simulink model "plant1_noObserver"  (R2015a)
settings: Solver=ode45  StartTime=0.0  StopTime=10.0  RelTol=1e-3
values from neighbouring files (symbols this model uses):
  A = [2.15382349002 0.214572825654 1.88950096566 -0.29867853041 0.113062196229 -1.01325242733 0.619436209547 2.86203861181 4.48591725582 -0.687413149535 3.93984391159 1.51814076611 ... (36 elements, 6x6)]    [De2.mat]    (also in main_elca.m = [   -2.1     0.3     0.5     0.9; main_elca_nonsquare.m = [-31.31 0 -2.833e4;0 -10.25 8001;1 -1 0]; main_elca_siso.m = [-31.31 0 -2.833e4;0 -10.25 8001;1 -1 0]; main_elca_siso_conference.m = [-31.31 0 -2.833e4;0 -10.25 8001;1 -1 0])
  B = [-3.59754701628 1.03900107164 -0.0588288788819 1.91030576689 -0.469593029649 2.39038747798 -2.63971513379 2.37119746965 -0.382769327239 -1.07761123079 -0.524364953631 2.34772297005 ... (18 elements, 6x3)]    [De2.mat]    (also in main_elca.m = [   1   -0.4; main_elca_nonsquare.m = [28.06 0 0]'; main_elca_siso.m = [28.06 0 0]'; main_elca_siso_conference.m = [28.06;0;0])
  C = [2.23974909489  -2.89672334174  -0.970355173176  -2.60836731796  -0.958327072966  -1.82597470965; -0.233950036489  3.17111373121  -0.953917376412  0.311760155602  0.255404296822  2.81333280658]    [De2.mat]    (also in main_elca.m = [2  -2  -1   4; main_elca_nonsquare.m = [1 0 0]; main_elca_siso.m = [1 0 0]; main_elca_siso_conference.m = [1 0 0])
  D = [0  0  0; 0  0  0]    [De2.mat]    (also in main_c.m = zeros(p,m); main_elca.m = zeros(p,m); main_elca_nonsquare.m = zeros(p,m); main_elca_siso.m = zeros(p,m))
  Ec = -inv(R_bar)*( ( C - D*Kc )*inv( A - B*Kc )*B - D )'*Qc    [TZOCS.m]    (also in main_c.m = -inv(R_bar)*( ( C_aug - D_aug*Kc )*inv( A_aug - B_aug*Kc )*B; main_elca.m = -inv(R_bar)*( ( C_aug - D_aug*Kc )*inv( A_aug - B_aug*Kc )*B; main_elca_nonsquare.m = -inv(R_bar)*( ( C_aug - D_aug*Kc )*inv( A_aug - B_aug*Kc )*B; main_elca_siso.m = -inv(R_bar)*( ( C_aug - D_aug*Kc )*inv( A_aug - B_aug*Kc )*B)
  eta = 0.532094499421    [eta value.mat]    (also in eta_value.mat = [-2.43750362486  -7.92336865107; -8.9760065871  -9.529746909; generate_eta.m = (1*randn(p,p)); main_c.m = 10*eta; main_elca_nonsquare.m = eye(1))
  Kc1 = Kc(:,1:n)    [main_c.m]    (also in main_elca.m; main_elca_nonsquare.m; main_elca_siso.m; main_elca_siso_conference.m)
  Kc2 = Kc(:,n+1:end)    [main_c.m]    (also in main_elca.m; main_elca_nonsquare.m; main_elca_siso.m; main_elca_siso_conference.m)
  Kd_1 = Kd(1,1)    [main_c.m]    (also in main_elca.m; main_elca_nonsquare.m; main_elca_siso.m; main_elca_siso_conference.m)
  Ki_1 = Ki(1,1)    [main_c.m]    (also in main_elca.m; main_elca_nonsquare.m; main_elca_siso.m; main_elca_siso_conference.m)
  Kp_1 = Kp(1,1)    [main_c.m]    (also in main_elca.m; main_elca_nonsquare.m; main_elca_siso.m; main_elca_siso_conference.m)
settings Model: Creator=Elca  LastModifiedBy=Elca

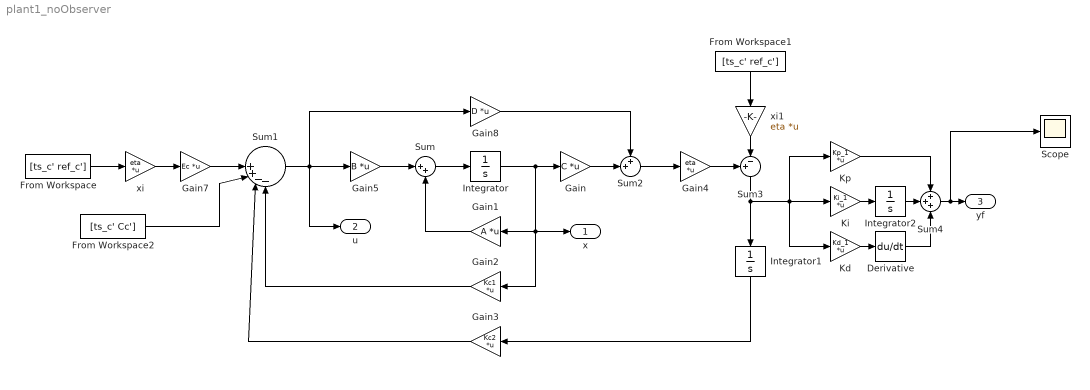
== system plant1_noObserver ==
  Derivative : Derivative
  From Workspace : FromWorkspace  VariableName=[ts_c' ref_c']  SampleTime=0
  From Workspace1 : FromWorkspace  VariableName=[ts_c' ref_c']  SampleTime=0
  From Workspace2 : FromWorkspace  VariableName=[ts_c' Cc']  SampleTime=0
  Gain : Gain  Gain=C  Multiplication=Matrix(K*u)
  Gain1 : Gain  Gain=A  Multiplication=Matrix(K*u)
  Gain2 : Gain  Gain=Kc1  Multiplication=Matrix(K*u)
  Gain3 : Gain  Gain=Kc2  Multiplication=Matrix(K*u)
  Gain4 : Gain  Gain=eta  Multiplication=Matrix(K*u)
  Gain5 : Gain  Gain=B  Multiplication=Matrix(K*u)
  Gain7 : Gain  Gain=Ec  Multiplication=Matrix(K*u)
  Gain8 : Gain  Gain=D  Multiplication=Matrix(K*u)
  Integrator : Integrator
  Integrator1 : Integrator
  Integrator2 : Integrator
  Kd : Gain  Gain=Kd_1  Multiplication=Matrix(K*u)
  Ki : Gain  Gain=Ki_1  Multiplication=Matrix(K*u)
  Kp : Gain  Gain=Kp_1  Multiplication=Matrix(K*u)
  Scope : Scope
  Sum : Sum  Inputs=|++
  Sum1 : Sum  Inputs=|||++--
  Sum2 : Sum  Inputs=++|
  Sum3 : Sum  Inputs=+-|
  Sum4 : Sum  Inputs=+++
  xi : Gain  Gain=eta  Multiplication=Matrix(K*u)
  xi1 : Gain  Gain=eta  Multiplication=Matrix(K*u)
  x : Outport
  u : Outport  Port=2
  yf : Outport  Port=3
  wires:
  Gain7/1 -> Sum1/1
  Integrator/1 -> Gain2/1, x/1, Gain1/1, Gain/1
  Sum2/1 -> Gain4/1
  Gain/1 -> Sum2/2
  Gain8/1 -> Sum2/1
  Sum1/1 -> Gain8/1, u/1, Gain5/1
  Sum/1 -> Integrator/1
  Gain1/1 -> Sum/2
  Gain5/1 -> Sum/1
  From Workspace/1 -> xi/1
  Integrator1/1 -> Gain3/1
  From Workspace2/1 -> Sum1/2
  Gain2/1 -> Sum1/4
  Gain3/1 -> Sum1/3
  Gain4/1 -> Sum3/1
  From Workspace1/1 -> xi1/1
  Sum3/1 -> Kd/1, Kp/1, Ki/1, Integrator1/1
  xi/1 -> Gain7/1
  xi1/1 -> Sum3/2
  Kd/1 -> Derivative/1
  Kp/1 -> Sum4/1
  Integrator2/1 -> Sum4/2
  Sum4/1 -> Scope/1, yf/1
  Derivative/1 -> Sum4/3
  Ki/1 -> Integrator2/1
